simulink model "ControllerDesign_STD"  (R2017b)
settings: Solver=ode4  StartTime=0.0  StopTime=10  FixedStep=0.01  RelTol=1e-3
undefined symbols (not defined in the file or in its folder): Linmod
settings Model: Creator=zht  LastModifiedBy=One

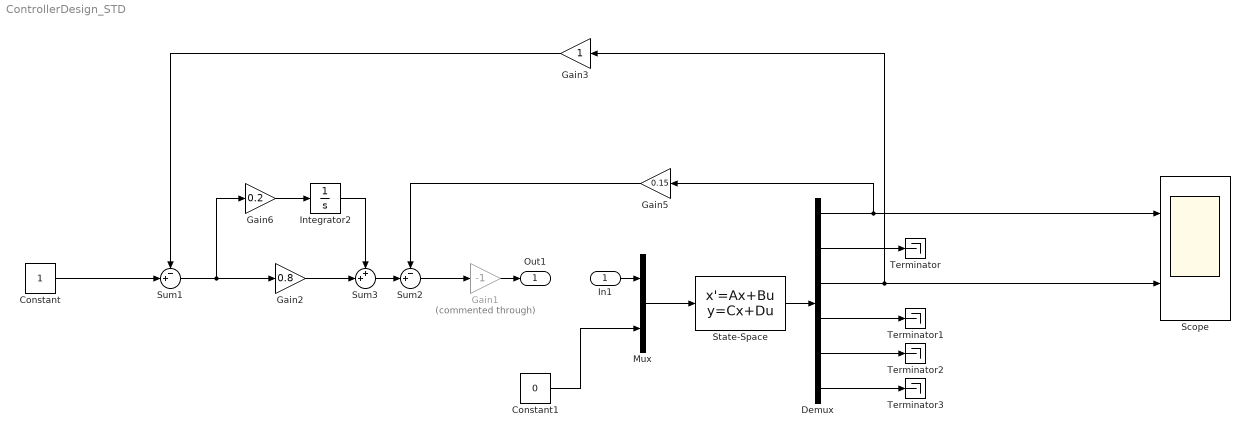
== system ControllerDesign_STD ==
  In1 : Inport
  Constant : Constant
  Constant1 : Constant  Value=0
  Demux : Demux  Outputs=6
  Gain1 : Gain  Commented=through  Gain=-1
  Gain2 : Gain  Gain=0.8
  Gain3 : Gain
  Gain5 : Gain  Gain=0.15
  Gain6 : Gain  Gain=0.2
  Integrator2 : Integrator
  Mux : Mux  Inputs=2
  Scope : Scope  NumInputPorts=2
  State-Space : StateSpace  A=Linmod.Lon_4b.A  B=Linmod.Lon_4b.B  C=Linmod.Lon_4b.C  D=Linmod.Lon_4b.D  InitialCondition=0
  Sum1 : Sum  Inputs=-+|
  Sum2 : Sum  Inputs=-+|
  Sum3 : Sum  Inputs=++|
  Terminator{,1..3} (4 alike) : Terminator
  Out1 : Outport
  wires:
  Constant1/1 -> Mux/2
  State-Space/1 -> Demux/1
  Demux/2 -> Terminator/1
  Demux/4 -> Terminator1/1
  Demux/5 -> Terminator2/1
  Demux/6 -> Terminator3/1
  Demux/1 -> Gain5/1, Scope/1
  Demux/3 -> Gain3/1, Scope/2
  Sum1/1 -> Gain6/1, Gain2/1
  Constant/1 -> Sum1/2
  Gain5/1 -> Sum2/1
  Gain3/1 -> Sum1/1
  Sum2/1 -> Gain1/1
  Gain6/1 -> Integrator2/1
  Gain2/1 -> Sum3/2
  Sum3/1 -> Sum2/2
  Integrator2/1 -> Sum3/1
  Mux/1 -> State-Space/1
  Gain1/1 -> Out1/1
  In1/1 -> Mux/1
